simulink model "Ultra_Local_Model_1_Ali37_MIMO_04_WMR_09"  (R2017b)
settings: Solver=ode45  StartTime=0.0  StopTime=500  RelTol=1e-3  EnableMultiTasking=on
InitFcn:
  | Cons_Ali_Mimo_04_WMR_09
values from neighbouring files (symbols this model uses):
  B = 1e0*eye(n)    [Cons_AMFC_Quad_New_01.m]    (also in Cons_Ali_Mimo_04_Quad_Observer.m; Cons_Ali_Mimo_04_WMR_09.m = 1*eye(n))
  BBT_inv = ((B'*B)^(-1))*B'    [Cons_AMFC_Quad_New_01.m]    (also in Cons_Ali_Mimo_04_Quad_Observer.m; Cons_Ali_Mimo_04_WMR_09.m)
  Cv = 0.1    [Cons_Ali_Mimo_04_WMR_09.m]
  Cw = 0.1    [Cons_Ali_Mimo_04_WMR_09.m]
  gamma_0 = 1e-0*diag([1e-3*ones(3,1);1e-0*ones(3,1)])    [Cons_AMFC_Quad_New_01.m]    (also in Cons_Ali_Mimo_04_Quad_Observer.m = 1e-0*diag([1e-3*ones(6,1);1e-3*ones(2,1);1e-0*ones(4,1)]); Cons_Ali_Mimo_04_WMR_09.m = 1e-1*diag([1e-3*ones(2,1);1e0*ones(2,1)]))
  gamma_1 = 1e+2*diag([1e-3*ones(3,1);1e-0*ones(3,1)])    [Cons_AMFC_Quad_New_01.m]    (also in Cons_Ali_Mimo_04_Quad_Observer.m = 1e+1*diag([1e-3*ones(6,1);1e-3*ones(2,1);1e-0*ones(4,1)]); Cons_Ali_Mimo_04_WMR_09.m = 1e2*diag([1e-3*ones(2,1);1e0*ones(2,1)]))
  J = 1.2416e-3 * diag([1 1 2])    [Cons_AMFC_Quad_New_01.m]    (also in Cons_Ali_Mimo_04_Quad_Observer.m; Cons_Ali_Mimo_04_WMR_09.m = 0.01)
  k1 = 1    [Cons_AMFC_Quad_New_01.m]    (also in Cons_Ali_Mimo_04_Quad_Observer.m; Cons_Ali_Mimo_04_WMR_09.m)
  k2 = 0.1    [Cons_AMFC_Quad_New_01.m]    (also in Cons_Ali_Mimo_04_Quad_Observer.m = 1; Cons_Ali_Mimo_04_WMR_09.m = 1)
  L0 = 0.1    [Cons_Ali_Mimo_04_WMR_09.m]
  m = 6    [Cons_AMFC_Quad_New_01.m]    (also in Cons_Ali_Mimo_04_Quad_Observer.m = 12; Cons_Ali_Mimo_04_WMR_09.m = 4)
  M = 2.95    [Cons_AMFC_Quad_New_01.m]    (also in Cons_Ali_Mimo_04_Quad_Observer.m; Cons_Ali_Mimo_04_WMR_09.m = 1)
  n = 6    [Cons_AMFC_Quad_New_01.m]    (also in Cons_Ali_Mimo_04_Quad_Observer.m = 12; Cons_Ali_Mimo_04_WMR_09.m = 4)
  nd = 2    [Cons_Ali_Mimo_04_WMR_09.m]
  Q = 1e-1*eye(n)    [Cons_AMFC_Quad_New_01.m]    (also in Cons_Ali_Mimo_04_Quad_Observer.m = 1e-2*eye(n); Cons_Ali_Mimo_04_WMR_09.m)
  R = 1e+0*eye(m)    [Cons_AMFC_Quad_New_01.m]    (also in Cons_Ali_Mimo_04_Quad_Observer.m; Cons_Ali_Mimo_04_WMR_09.m = 1*eye(m))
  R0 = 0.1    [Cons_Ali_Mimo_04_WMR_09.m]
  rho_0 = 1e-0    (= 1)    [Cons_AMFC_Quad_New_01.m]    (also in Cons_Ali_Mimo_04_Quad_Observer.m = 0.001; Cons_Ali_Mimo_04_WMR_09.m = 0.0001)
  rho_1 = 1e-0    (= 1)    [Cons_AMFC_Quad_New_01.m]    (also in Cons_Ali_Mimo_04_Quad_Observer.m = 0.001; Cons_Ali_Mimo_04_WMR_09.m = 0.001)
settings Model: SimulationMode=rapid-accelerator  Creator=hp  LastModifiedBy=ali.safaei
settings DataIOCC: LimitDataPoints=on  SaveFormat=Array
settings OptimizationCC: LifeSpan=inf
settings DebuggingCC: UnderspecifiedInitializationDetection=Classic  MergeDetectMultiDrivingBlocksExec=none  SolverPrmCheckMsg=warning  SFUnexpectedBacktrackingDiag=warning  SFNoUnconditionalDefaultTransitionDiag=warning  SFExecutionAtInitializationDiag=none
settings HardwareCC: ProdBitPerPointer=32  ProdBitPerSizeT=32  ProdBitPerPtrDiffT=32  ProdLargestAtomicFloat=None  ProdIntDivRoundTo=Undefined  ProdEndianess=Unspecified  ProdWordSize=32  ProdHWDeviceType=32-bit Generic
settings ModelReferenceCC: PropagateSignalLabelsOutOfModel=off
settings CodeAppCC: StateflowObjectComments=on
settings GRTTargetCC: TargetLangStandard=C89/C90 (ANSI)  GeneratePreprocessorConditionals=Disable all
settings ConfigComp: CovMetricSettings=dw  CovHtmlReporting=on  CovSaveCumulativeToWorkspaceVar=on  CovSaveSingleToWorkspaceVar=on  CovExternalEMLEnable=off

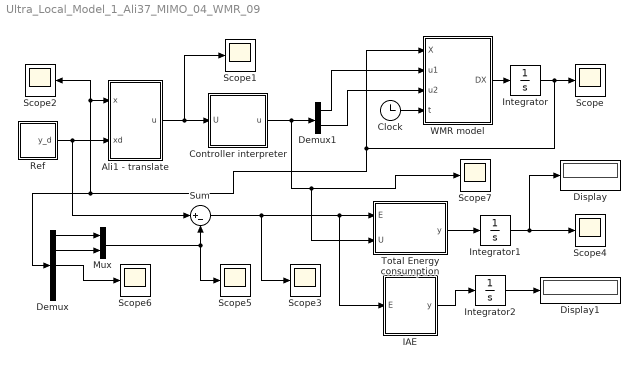
== system Ultra_Local_Model_1_Ali37_MIMO_04_WMR_09 ==
  Ali1 - translate : Subsystem
  Clock : Clock
  Controller interpreter : MATLAB Function  TreatAsAtomicUnit=on
  Demux : Demux  Outputs=5
  Demux1 : Demux  Outputs=2
  Display : Display
  Display1 : Display
  IAE : MATLAB Function  TreatAsAtomicUnit=on
  Integrator : Integrator  InitialCondition=[0;0;0;0;0]
  Integrator1 : Integrator
  Integrator2 : Integrator
  Mux : Mux  Inputs=2
  Ref : Subsystem
  Scope{,1..7} (8 alike) : Scope
  Sum : Sum  Inputs=|+-
  Total Energy consumption : MATLAB Function  TreatAsAtomicUnit=on
  WMR model : MATLAB Function  TreatAsAtomicUnit=on
  wires:
  WMR model/1(DX) -> Integrator/1
  Integrator/1 -> Scope/1, WMR model/1(X), Scope2/1, Ali1 - translate/1(x), Demux/1
  Integrator1/1 -> Display/1, Scope4/1
  Total Energy consumption/1(y) -> Integrator1/1
  Ref/1(y_d) -> Ali1 - translate/2(xd), Sum/1
  Integrator2/1 -> Display1/1
  Sum/1 -> Total Energy consumption/1(E), IAE/1(E), Scope3/1
  IAE/1(y) -> Integrator2/1
  Demux/1 -> Mux/1
  Demux/2 -> Mux/2
  Mux/1 -> Scope5/1, Sum/2
  Ali1 - translate/1(u) -> Controller interpreter/1(U), Scope1/1
  Demux/3 -> Scope6/1
  Clock/1 -> WMR model/4(t)
  Demux1/1 -> WMR model/2(u1)
  Demux1/2 -> WMR model/3(u2)
  Controller interpreter/1(u) -> Scope7/1, Total Energy consumption/2(U), Demux1/1

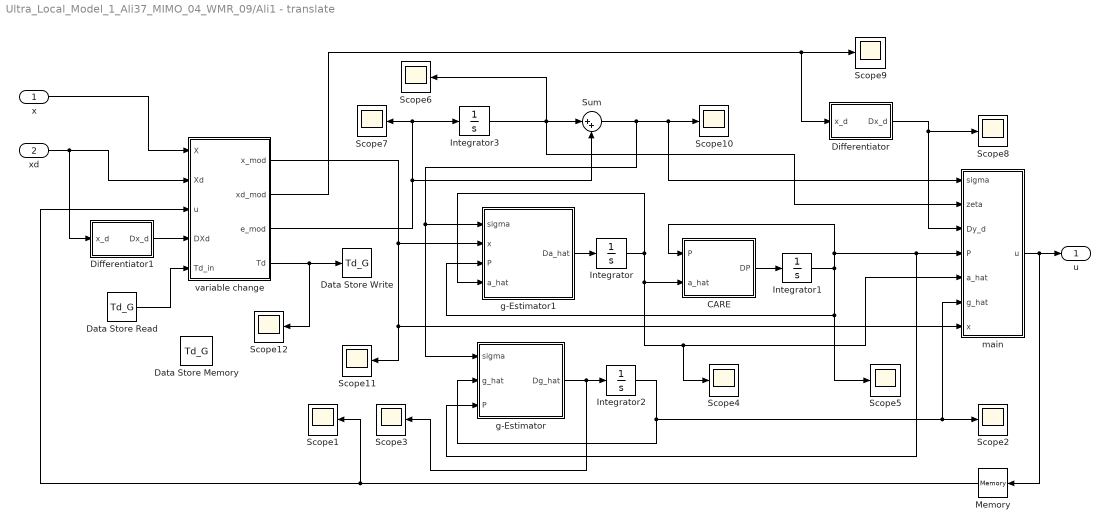
== system Ultra_Local_Model_1_Ali37_MIMO_04_WMR_09/Ali1 - translate ==
  x : Inport
  xd : Inport  Port=2
  CARE : MATLAB Function  TreatAsAtomicUnit=on
  Data Store Memory : DataStoreMemory  DataStoreName=Td_G  ReadBeforeWriteMsg=warning  WriteAfterWriteMsg=warning  WriteAfterReadMsg=warning  ShowAdditionalParam=off
  Data Store Read : DataStoreRead  DataStoreName=Td_G
  Data Store Write : DataStoreWrite  DataStoreName=Td_G
  Differentiator : Subsystem
  Differentiator1 : Subsystem
  Integrator : Integrator  InitialCondition=zeros(n)
  Integrator1 : Integrator  InitialCondition=eye(n)
  Integrator2 : Integrator  InitialCondition=zeros(n,1)
  Integrator3 : Integrator  InitialCondition=zeros(n,1)
  Memory : Memory  InitialCondition=zeros(m,1)
  Scope{1..12} (12 alike) : Scope
  Sum : Sum  Inputs=|++
  g-Estimator : MATLAB Function  TreatAsAtomicUnit=on
  g-Estimator1 : MATLAB Function  TreatAsAtomicUnit=on
  main : MATLAB Function  TreatAsAtomicUnit=on
  variable change : MATLAB Function  TreatAsAtomicUnit=on
  u : Outport
  wires:
  g-Estimator/1(Dg_hat) -> Scope3/1, Integrator2/1
  Integrator2/1 -> g-Estimator/2(g_hat), Scope2/1, main/6(g_hat)
  variable change/3(e_mod) -> Sum/2, Scope7/1, Integrator3/1
  Integrator3/1 -> main/2(zeta), Scope6/1, Sum/1
  variable change/1(x_mod) -> Scope11/1, main/7(x), g-Estimator1/2(x)
  g-Estimator1/1(Da_hat) -> Integrator/1
  Differentiator/1(Dx_d) -> Scope8/1, main/3(Dy_d)
  Sum/1 -> main/1(sigma), Scope10/1, g-Estimator/1(sigma), g-Estimator1/1(sigma)
  Integrator1/1 -> g-Estimator/3(P), main/4(P), CARE/1(P), Scope5/1, g-Estimator1/3(P)
  Integrator/1 -> main/5(a_hat), Scope4/1, CARE/2(a_hat), g-Estimator1/4(a_hat)
  x/1 -> variable change/1(X)
  main/1(u) -> u/1, Memory/1
  Memory/1 -> variable change/3(u), Scope1/1
  xd/1 -> variable change/2(Xd), Differentiator1/1(x_d)
  variable change/2(xd_mod) -> Differentiator/1(x_d), Scope9/1
  CARE/1(DP) -> Integrator1/1
  Differentiator1/1(Dx_d) -> variable change/4(DXd)
  Data Store Read/1 -> variable change/5(Td_in)
  variable change/4(Td) -> Data Store Write/1, Scope12/1

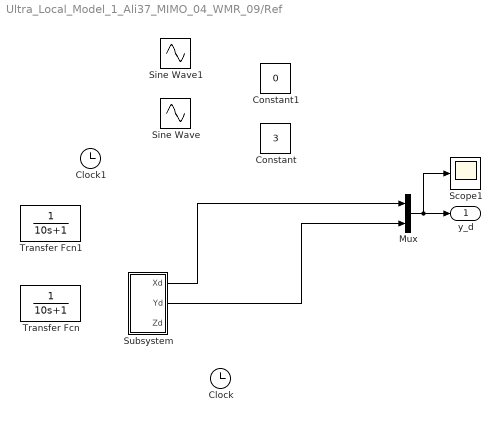
== system Ultra_Local_Model_1_Ali37_MIMO_04_WMR_09/Ref ==
  Clock : Clock
  Clock1 : Clock
  Constant : Constant  Value=3
  Constant1 : Constant  Value=0
  Mux : Mux  Inputs=2
  Scope1 : Scope
  Sine Wave : Sin  Amplitude=5  SampleTime=0
  Sine Wave1 : Sin  Amplitude=5  Phase=pi/2  SampleTime=0
  Subsystem : Subsystem
  Transfer Fcn : TransferFcn  Denominator=[10 1]
  Transfer Fcn1 : TransferFcn  Denominator=[10 1]
  y_d : Outport
  wires:
  Mux/1 -> Scope1/1, y_d/1
  Subsystem/2(Yd) -> Mux/2
  Subsystem/1(Xd) -> Mux/1

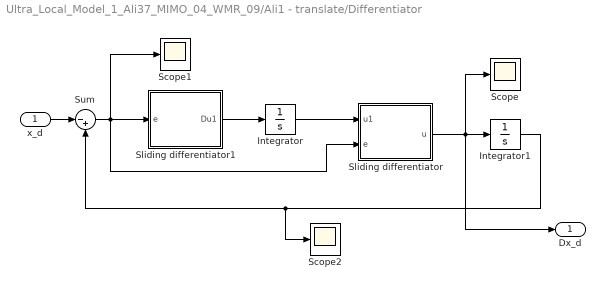
== system Ultra_Local_Model_1_Ali37_MIMO_04_WMR_09/Ali1 - translate/Differentiator ==
  x_d : Inport
  Integrator : Integrator  InitialCondition=zeros(n,1)
  Integrator1 : Integrator  InitialCondition=zeros(n,1)
  Scope : Scope
  Scope1 : Scope
  Scope2 : Scope
  Sliding differentiator : MATLAB Function  TreatAsAtomicUnit=on
  Sliding differentiator1 : MATLAB Function  TreatAsAtomicUnit=on
  Sum : Sum  Inputs=|-+
  Dx_d : Outport
  wires:
  Sliding differentiator1/1(Du1) -> Integrator/1
  Integrator/1 -> Sliding differentiator/1(u1)
  x_d/1 -> Sum/1
  Sum/1 -> Scope1/1, Sliding differentiator/2(e), Sliding differentiator1/1(e)
  Integrator1/1 -> Scope2/1, Sum/2
  Sliding differentiator/1(u) -> Dx_d/1, Scope/1, Integrator1/1

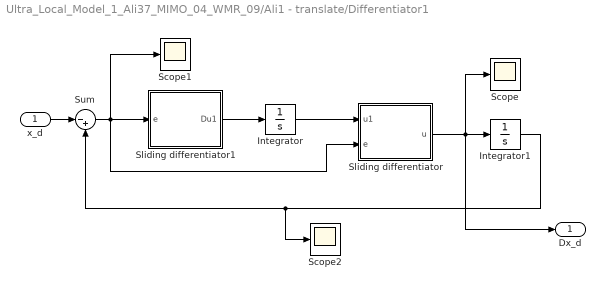
== system Ultra_Local_Model_1_Ali37_MIMO_04_WMR_09/Ali1 - translate/Differentiator1 ==
  x_d : Inport
  Integrator : Integrator  InitialCondition=zeros(nd,1)
  Integrator1 : Integrator  InitialCondition=zeros(nd,1)
  Scope : Scope
  Scope1 : Scope
  Scope2 : Scope
  Sliding differentiator : MATLAB Function  TreatAsAtomicUnit=on
  Sliding differentiator1 : MATLAB Function  TreatAsAtomicUnit=on
  Sum : Sum  Inputs=|-+
  Dx_d : Outport
  wires:
  Sliding differentiator1/1(Du1) -> Integrator/1
  Integrator/1 -> Sliding differentiator/1(u1)
  x_d/1 -> Sum/1
  Sum/1 -> Scope1/1, Sliding differentiator/2(e), Sliding differentiator1/1(e)
  Integrator1/1 -> Scope2/1, Sum/2
  Sliding differentiator/1(u) -> Dx_d/1, Scope/1, Integrator1/1

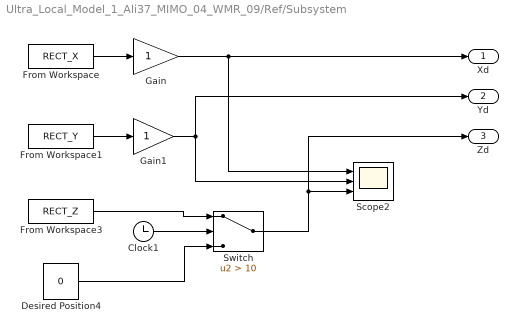
== system Ultra_Local_Model_1_Ali37_MIMO_04_WMR_09/Ref/Subsystem ==
  Clock1 : Clock
  Desired Position4 : Constant  Value=0  VectorParams1D=off
  From Workspace : FromWorkspace  VariableName=RECT_X  SampleTime=0
  From Workspace1 : FromWorkspace  VariableName=RECT_Y  SampleTime=0
  From Workspace3 : FromWorkspace  VariableName=RECT_Z  SampleTime=0
  Gain : Gain
  Gain1 : Gain
  Scope2 : Scope  NumInputPorts=3
  Switch : Switch  Criteria=u2 > Threshold  Threshold=10
  Xd : Outport
  Yd : Outport  Port=2
  Zd : Outport  Port=3
  wires:
  From Workspace/1 -> Gain/1
  From Workspace1/1 -> Gain1/1
  Clock1/1 -> Switch/2
  Switch/1 -> Zd/1, Scope2/3
  From Workspace3/1 -> Switch/1
  Desired Position4/1 -> Switch/3
  Gain/1 -> Scope2/1, Xd/1
  Gain1/1 -> Yd/1, Scope2/2

== matlab function Ultra_Local_Model_1_Ali37_MIMO_04_WMR_09/IAE ==
  data: E input; y output
function y = fcn(E)

Ea = abs(E(1:2));
%Qa = 1*eye(2);
y = sum(Ea); %Ea' * Qa * Ea;

end

== matlab function Ultra_Local_Model_1_Ali37_MIMO_04_WMR_09/WMR model ==
  data: X input; u1 input; DX output; u2 input; t input; Cv parameter; Cw parameter; M parameter; J parameter; R0 parameter; L0 parameter
function DX = fcn(X,u1,u2,t,Cv,Cw,M,J,R0,L0)

x = X(1);
y = X(2);
T = X(3);
v = X(4);
w = X(5);

T1 = 0.01 * u1; 
T2 = 0.01 * u2; 

F = (1/R0)*(T1+T2);
Tau = (L0/R0)*(T1-T2);

Dv = (F - Cv*v + (1*sin(1*t)))/M ;
Dw = (Tau - Cw*w + (1*sin(1*t)))/J ;

Dx = v*cos(T);
Dy = v*sin(T);
DT = w;

DX = [Dx Dy DT Dv Dw]';

end

== matlab function Ultra_Local_Model_1_Ali37_MIMO_04_WMR_09/Ali1 - translate/Differentiator/Sliding differentiator ==
  data: u output; u1 input; e input; n parameter; k1 parameter
function u = fcn(u1,e,n,k1)

b=k1;

ABS = zeros(n,1);
for i=1:n
    if e(i)>0
        ABS(i) = e(i);
    else
        ABS(i) = -e(i);
    end
end
SGN = e ./ (ABS + 0.01);

u = u1 - b*(ABS.^0.5).*SGN;

end

== matlab function Ultra_Local_Model_1_Ali37_MIMO_04_WMR_09/Ali1 - translate/Differentiator/Sliding differentiator1 ==
  data: Du1 output; e input; n parameter; k2 parameter
function Du1 = fcn(e,n,k2)

a=k2;

ABS = zeros(n,1);
for i=1:n
    if e(i)>0
        ABS(i) = e(i);
    else
        ABS(i) = -e(i);
    end
end
SGN = e ./ (ABS + 0.01);

Du1 = - a*SGN;

end

== matlab function Ultra_Local_Model_1_Ali37_MIMO_04_WMR_09/Ali1 - translate/g-Estimator ==
  data: sigma input; g_hat input; P input; rho_1 parameter; gamma_1 parameter; Dg_hat output
function Dg_hat = fcn(sigma,g_hat,P,rho_1,gamma_1)

Dg_hat = - gamma_1 * P * sigma - rho_1 * gamma_1 * g_hat;

end

== matlab function Ultra_Local_Model_1_Ali37_MIMO_04_WMR_09/Ali1 - translate/g-Estimator1 ==
  data: sigma input; x input; P input; rho_0 parameter; gamma_0 parameter; Da_hat output; a_hat input
function Da_hat = fcn(sigma,x,P,rho_0,gamma_0,a_hat)

DVa_hat = - gamma_0 * P * diag(sigma) * (x - sigma) - rho_0 * gamma_0 * diag(a_hat);
Da_hat = diag(DVa_hat);

end

== matlab function Ultra_Local_Model_1_Ali37_MIMO_04_WMR_09/Ali1 - translate/main ==
  data: sigma input; zeta input; u output; Dy_d input; R parameter; P input; a_hat input; B parameter; g_hat input; x input; Q parameter; BBT_inv parameter; n parameter
function u = fcn(sigma,zeta,Dy_d,R,P,a_hat,B,g_hat,x,Q,BBT_inv,n)

u1 = (1/2) * R * B' * P * sigma;
u2 = BBT_inv * (Dy_d - a_hat*x + (eye(n) + 2*(P^(-1)*Q) + a_hat)*sigma - g_hat - zeta) - (3/4) * R * B' * P * sigma;

u = u1 + u2;

end

== matlab function Ultra_Local_Model_1_Ali37_MIMO_04_WMR_09/Ali1 - translate/variable change ==
  data: X input; Xd input; x_mod output; u input; DXd input; xd_mod output; e_mod output; Td_in input; Thresh parameter; Td output
function [x_mod,xd_mod,e_mod,Td] = fcn(X,Xd,u,DXd,Td_in,Thresh)

T = X(3);

Td = Td_in;
if (abs(DXd(1))+abs(DXd(2))) > (1*Thresh)
    y_Err = (Xd(2)-X(2));
    x_Err = (Xd(1)-X(1));
    XS = (y_Err/x_Err);
    Td = atan(XS); 
    if abs(Td)>1.5
        Td = abs(Td);
    end
end

Pos = X(1)*cos(T) + X(2)*sin(T);
Posd = Xd(1)*cos(T) + Xd(2)*sin(T);

x_mod = [Pos;T;X(4);X(5)];
xd_mod = [Posd;Td;u(1);u(2)]; 

e_mod = xd_mod - x_mod;

end

== matlab function Ultra_Local_Model_1_Ali37_MIMO_04_WMR_09/Controller interpreter ==
  data: u output; U input
function u = fcn(U)

U1 = U(3);
U2 = U(4); 

u1 = 0.5 * (U1+U2);
u2 = 0.5 * (U1-U2);

u = [u1;u2];

end

== matlab function Ultra_Local_Model_1_Ali37_MIMO_04_WMR_09/Total Energy consumption ==
  data: E input; y output; U input
function y = fcn(E,U)

Ep = E(1:2);
Up = U(1:2);
Qe = 1*eye(2);
Re = 1*eye(2);
y = Ep' * Qe * Ep + Up' * Re * Up;

end

== matlab function Ultra_Local_Model_1_Ali37_MIMO_04_WMR_09/Ali1 - translate/CARE ==
  data: P input; a_hat input; B parameter; R parameter; DP output; Q parameter
function DP = fcn(P,a_hat,B,R,Q)

DP = a_hat*P + P*a_hat' - P*B*R*B'*P + 2*Q;

end

== matlab function Ultra_Local_Model_1_Ali37_MIMO_04_WMR_09/Ali1 - translate/Differentiator1/Sliding differentiator ==
  data: u output; u1 input; e input; nd parameter; k1 parameter
function u = fcn(u1,e,nd,k1)

b=10;

ABS = zeros(nd,1);
for i=1:nd
    if e(i)>0
        ABS(i) = e(i);
    else
        ABS(i) = -e(i);
    end
end
SGN = e ./ (ABS + 0.01);

u = u1 - b*(ABS.^0.5).*SGN;

end

== matlab function Ultra_Local_Model_1_Ali37_MIMO_04_WMR_09/Ali1 - translate/Differentiator1/Sliding differentiator1 ==
  data: Du1 output; e input; nd parameter; k2 parameter
function Du1 = fcn(e,nd,k2)

a=k2;

ABS = zeros(nd,1);
for i=1:nd
    if e(i)>0
        ABS(i) = e(i);
    else
        ABS(i) = -e(i);
    end
end
SGN = e ./ (ABS + 0.01);

Du1 = - a*SGN;

end
